simulink model "MicroMouseTemplate2"  (R2023a)
settings: Solver=FixedStepAuto  StartTime=0.0  StopTime=10.0  RelTol=1e-3  EnableMultiTasking=on
undefined symbols (not defined in the file): samplingTime
settings Model: STM32="{\"DigitalPortWrite\":[{\"ID\":\"MicroMouseTemplate:84:3\"},{\"ID\":\"MicroMouseTemplate:84:4\"},{\"ID\":\"MicroMouseTemplate:84:5\"},{\"ID\":\"MicroMouseTemplate:84:6\"},{\"ID\":\"MicroMouseTemplate:84:7\"},{\"ID\":\"MicroMouseTemplate:84:8\"},{\"ID\":\"MicroMouseTemplate:84:9\"},{\"ID\":\"MicroMouseTemplate:84:10\"},{\"ID\":\"MicroMouseTemplate:160:19\"},{\"ID\":\"MicroMouseTemplate:2479:4\"},{\"ID\":\"MicroMouseTemplate:2479:6\"},{\"ID\":\"MicroMouseTemplate:2479:7\"},{\"ID\":\"MicroMouseTemplate:2479:8\"},{\"ID\":\"MicroMouseTemplate2:84:3\"},{\"ID\":\"MicroMouseTemplate2:84:4\"},{\"ID\":\"MicroMouseTemplate2:84:5\"},{\"ID\":\"MicroMouseTemplate2:84:6\"},{\"ID\":\"MicroMouseTemplate2:84:7\"},{\"ID\":\"MicroMouseTemplate2:84:8\"},{\"ID\":\"MicroMouseTemplate2:84:9\"},{\"ID\":\"MicroMouseTemplate2:84:10\"},{\"ID\":\"MicroMouseTemplate2:160:19\"},{\"ID\":\"MicroMouseTemplate2:2479:4\"},{\"ID\":\"MicroMouseTemplate2:2479:6\"},{\"ID\":\"MicroMouseTemplate2:2479:7\"},{\"ID\":\"MicroMouseTemplate2:2479:8\"}],\"PWMOutput\":[{\"ID\":\"MicroMouseTemplate:160:24\"},{\"ID\":\"MicroMouseTemplate:160:25\"},{\"ID\":\"MicroMouseTemplate2:160:24\"},{\"ID\":\"MicroMouseTemplate2:160:25\"}],\"AnalogInput\":[{\"ID\":\"MicroMouseTemplate:2357:1\"},{\"ID\":\"MicroMouseTemplate2:2357:1\"}],\"DigitalPortRead\":[{\"ID\":\"MicroMouseTemplate:2483:3\"},{\"ID\":\"MicroMouseTemplate:2483:4\"},{\"ID\":\"MicroMouseTemplate2:2483:3\"},{\"ID\":\"MicroMouseTemplate2:2483:4\"}]}"  SimulationMode=external  ExtModeTrigDuration=10  Creator=JesseJabezArendse  LastModifiedBy=khanm
settings SolverCC: AllowMultiTaskInputOutput=on  AutoInsertRateTranBlk=on  InsertRTBMode=Never (minimum delay)
settings OptimizationCC: EnhancedBackFolding=on  PassReuseOutputArgsAs=Individual arguments  StateBitsets=on  DataBitsets=on  ZeroExternalMemoryAtStartup=off  ZeroInternalMemoryAtStartup=off  NoFixptDivByZeroProtection=on  MaxStackSize=64  OptimizeBlockOrder=speed  DifferentSizesBufferReuse=on  EfficientTunableParamExpr=on
settings DebuggingCC: MultiTaskCondExecSysMsg=none  ParameterOverflowMsg=none  ParameterPrecisionLossMsg=none  ParameterTunabilityLossMsg=error
settings HardwareCC: ProdBitPerPointer=32  ProdBitPerSizeT=32  ProdBitPerPtrDiffT=32  ProdLargestAtomicInteger=Long  ProdLargestAtomicFloat=Double  ProdWordSize=32  ProdLongLongMode=on  ProdHWDeviceType=ARM Compatible->ARM Cortex  TargetBitPerPointer=64  TargetBitPerSizeT=64  TargetBitPerPtrDiffT=64  TargetLongLongMode=on  TargetIntDivRoundTo=Zero  TargetEndianess=LittleEndian  TargetWordSize=64  TargetHWDeviceType=MATLAB Host
settings ModelReferenceCC: EnableParallelModelReferenceBuilds=on  ParallelModelReferenceMATLABWorkerInit=Copy Base Workspace  SupportModelReferenceSimTargetCustomCode=on
settings SFSimCC: MATLABDynamicMemAlloc=off  SimHardwareAcceleration=native
settings RTWCC: Description=Embedded Coder  SystemTargetFile=ert.tlc  HardwareBoard=STM32L4xx Based  TLCOptions=-p0 -aInlineSetEventsForThisBaseRateFcn=TLC_FALSE -aSuppressMultiTaskScheduler=TLC_FALSE -aRateBasedStepFcn=1  TemplateMakefile=ert_default_tmf  Toolchain=GNU Tools for ARM Embedded Processors  CodeExecutionProfiling=on  CodeProfilingInstrumentation=coarse
settings RTWCC: CustomHeaderCode=|
  | #include "MicroMouseProgramming\Core\Inc\IMU.h"
  | #include "MicroMouseProgramming\Core\Inc\CustomWhile.h"
  | #include "MicroMouseProgramming\Core\Inc\Motors.h"
settings RTWCC: CustomInclude=|
  | MicroMouseProgramming\Core\Inc\
  | MicroMouseProgramming\Core\Src\
settings RTWCC: CustomSource=|
  | MicroMouseProgramming\Core\Src\IMU.c
  | MicroMouseProgramming\Core\Src\CustomWhile.c
  | MicroMouseProgramming\Core\Src\Motors.c
settings CodeAppCC: ForceParamTrailComments=on  IgnoreCustomStorageClasses=off  OperatorAnnotations=on  SimulinkDataObjDesc=on  SFDataObjDesc=on  InsertBlockDesc=on
settings ERTTargetCC: CodeReplacementLibrary=ARM Cortex-M  SupportNonFinite=off  SupportComplex=off  ExtModeTransport=3  ExtModeStaticAlloc=on  ExtModeStaticAllocSize=2048  ExtModeMexFile=ext_xcp  ExtModeIntrfLevel=Level2 - Open

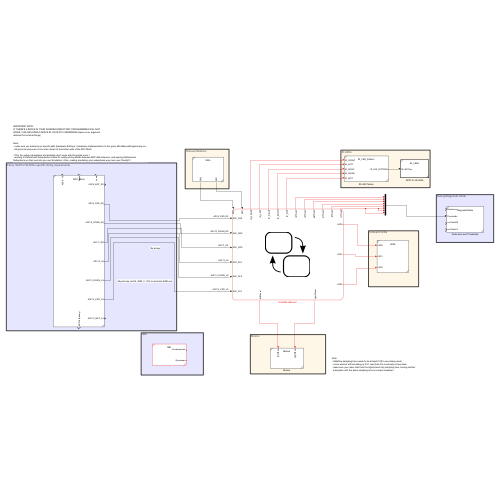
[thumbnail: Simulink's stored preview of the top-level diagram]
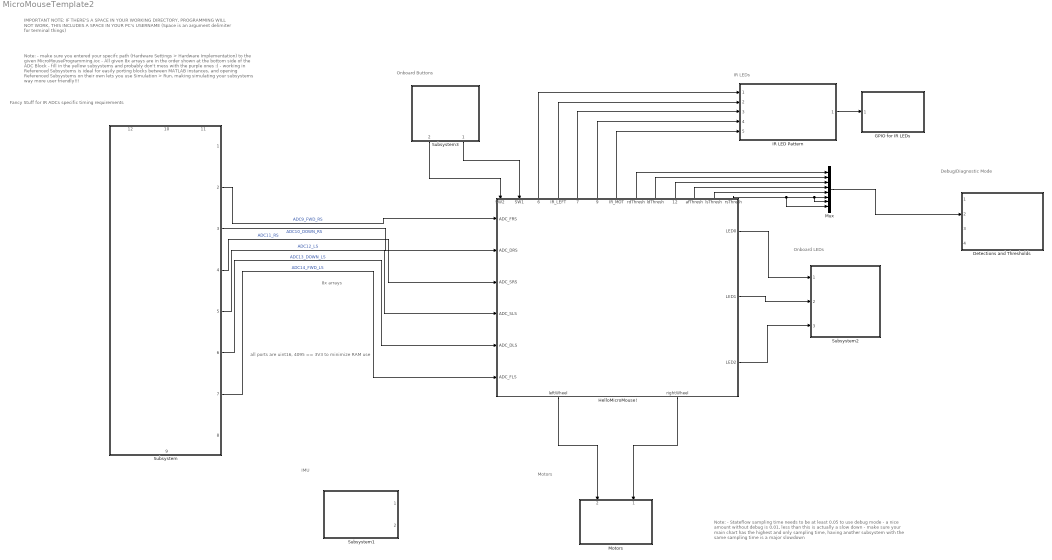
== system MicroMouseTemplate2 ==
  note: IMPORTANT NOTE:
      | IF THERE'S A SPACE IN YOUR WORKING DIRECTORY, PROGRAMMING WILL NOT WORK, THIS INCLUDES A SPACE IN YOUR PC's USERNAME (Space is an argument delimiter for terminal things)
  note: Note:
      | - make sure you entered your specifc path (Hardware Settings > Hardware Implementation) to the given MicroMouseProgramming.ioc
      | - All given 8x arrays are in the order shown at the bottom side of the ADC Block
      |
      | - fill in the yellow subsystems and probably don't mess with the purple ones :)
      | - working in Referenced Subsystems is ideal for easily porting blocks between MATLAB instances, and opening Referenced Subsystems on their own lets you use Simulation > Run, making simulating your subsystems way more user friendly!!!
  note: 8x arrays
  note: all ports are uint16, 4095 == 3V3 to minimize RAM use
  note: IMU
  note: Note:
      | - Stateflow sampling time needs to be at least 0.05 to use debug mode
      | - a nice amount without debug is 0.01, less than this is actually a slow down
      | - make sure your main chart has the highest and only sampling time, having another
      | subsystem with the same sampling time is a major slowdown
  note: Fancy Stuff for IR ADCs specific timing requirements
  note: IR LEDs
  note: Motors
  note: Onboard Buttons
  note: Onboard LEDs
  note: Debug/Diagnostic Mode
  Detections and Thresholds : Subsystem  ReferencedSubsystem=DiagnosticMode
  GPIO for IR LEDs : Subsystem  TreatAsAtomicUnit=on  SystemSampleTime=samplingTime  ReferencedSubsystem=IR_LEDs
  HelloMicroMouse! : Stateflow chart  TreatAsAtomicUnit=on
      settings: PortSchema="{\"entries\":[{\"content\":{\"sides\":[{\"content\":{\"connectorIds\":[\"In6\",\"In3\",\"In8\",\"In7\",\"In4\",\"In5\"]},\"type\":\"ConnectorPlacement.EquallySpacedRectSide\",\"uuid\":\"f52daa4f-6374-42e5-9ef1-0ccc99d09b58\"},{\"content\":{\"connectorIds\":[\"Out1\",\"Out4\",\"Out5\"],\"side\":\"RIGHT\"},\"type\":\"ConnectorPlacement.EquallySpacedRectSide\",\"uuid\":\"94b478cc-4dde-45c7-a588-77cf2b43cdb7\"},{\"content\":{\"connectorIds\":[\"In1\",\"In2\",\"Out6\",\"Out8\",\"Out7\",\"Out9\",\"Out16\",\"Out10\",\"Out11\",\"Out12\",\"Out13\",\"Out14\",\"Out15\"],\"side\":\"TOP\"},\"type\":\"ConnectorPlacement.EquallySpacedRectSide\",\"uuid\":\"afff2079-ea5c-423e-9722-09c3bbce433b\"},{\"content\":{\"connectorIds\":[\"Out2\",\"Out3\"],\"side\":\"BOTTOM\"},\"type\":\"ConnectorPlacement.EquallySpacedRectSide\",\"uuid\":\"94e93a1d-795d-41a3-b2d8-d520b2bf47ef\"}]},\"type\":\"ConnectorPlacement.EquallySpacedConnector\",\"uuid\":\"d4d35636-54af-48ac-af70-d56caef5e090\"}],\"packageUris\":[\"http://schema.mathworks.com/mf0/Connector/R2020b\"],\"version\":\"1.0\"}"
  IR LED Pattern : Subsystem  ReferencedSubsystem=IR_LED_Pattern
  Motors : Subsystem  ReferencedSubsystem=Motors
      settings: PortSchema="{\"entries\":[{\"content\":{\"sides\":[{\"content\":{},\"type\":\"ConnectorPlacement.EquallySpacedRectSide\",\"uuid\":\"c0768360-d607-41d7-924d-4f6c7a7c5513\"},{\"content\":{\"side\":\"RIGHT\"},\"type\":\"ConnectorPlacement.EquallySpacedRectSide\",\"uuid\":\"76549d19-b608-4a9d-9981-587ff77a2575\"},{\"content\":{\"connectorIds\":[\"In2\",\"In1\"],\"side\":\"TOP\"},\"type\":\"ConnectorPlacement.EquallySpacedRectSide\",\"uuid\":\"f7c4009a-c050-4e8b-9774-5a337efc0393\"}]},\"type\":\"ConnectorPlacement.EquallySpacedConnector\",\"uuid\":\"93b2f239-44e8-47ae-a398-357dc23e174c\"}],\"packageUris\":[\"http://schema.mathworks.com/mf0/Connector/R2020b\"],\"version\":\"1.0\"}"
  Mux : Mux  Inputs=8
  Subsystem : Subsystem  ReferencedSubsystem=ADC_Block
      settings: PortSchema="{\"entries\":[{\"content\":{\"sides\":[{\"content\":{},\"type\":\"ConnectorPlacement.EquallySpacedRectSide\",\"uuid\":\"be6b81d5-7a49-4e34-b35f-0c07892094fc\"},{\"content\":{\"connectorIds\":[\"Out1\",\"Out2\",\"Out3\",\"Out4\",\"Out5\",\"Out6\",\"Out7\",\"Out8\"],\"side\":\"RIGHT\"},\"type\":\"ConnectorPlacement.EquallySpacedRectSide\",\"uuid\":\"5e22590a-b7c0-4c63-8de4-8d81fd6c3849\"},{\"content\":{\"connectorIds\":[\"Out12\",\"Out10\",\"Out11\"],\"side\":\"TOP\"},\"type\":\"ConnectorPlacement.EquallySpacedRectSide\",\"uuid\":\"da97636e-cea0-4a10-8fe5-d807f9ee999f\"},{\"content\":{\"connectorIds\":[\"Out9\"],\"side\":\"BOTTOM\"},\"type\":\"ConnectorPlacement.EquallySpacedRectSide\",\"uuid\":\"a593d780-81a8-4730-a8bc-2bbf356cafe4\"}]},\"type\":\"ConnectorPlacement.EquallySpacedConnector\",\"uuid\":\"0bcac921-e51a-4437-9183-315712d0a8c2\"}],\"packageUris\":[\"http://schema.mathworks.com/mf0/Connector/R2020b\"],\"version\":\"1.0\"}"
  Subsystem1 : Subsystem  ReferencedSubsystem=IMU
  Subsystem2 : Subsystem  ReferencedSubsystem=LEDs
  Subsystem3 : Subsystem  ReferencedSubsystem=SWs
      settings: PortSchema="{\"entries\":[{\"content\":{\"sides\":[{\"content\":{},\"type\":\"ConnectorPlacement.EquallySpacedRectSide\",\"uuid\":\"525c1d33-3535-4f4c-aa7a-529c732595a4\"},{\"content\":{\"side\":\"RIGHT\"},\"type\":\"ConnectorPlacement.EquallySpacedRectSide\",\"uuid\":\"892b90bb-1dbb-40cd-aa67-d09788eff32d\"},{\"content\":{\"side\":\"TOP\"},\"type\":\"ConnectorPlacement.EquallySpacedRectSide\",\"uuid\":\"6623a0d6-78eb-4978-b109-dfe6d3d1ab9b\"},{\"content\":{\"connectorIds\":[\"Out2\",\"Out1\"],\"side\":\"BOTTOM\"},\"type\":\"ConnectorPlacement.EquallySpacedRectSide\",\"uuid\":\"a7ac3c79-7bca-470d-bb1f-b760bc3a3657\"}]},\"type\":\"ConnectorPlacement.EquallySpacedConnector\",\"uuid\":\"47292853-ce7e-4392-82cf-216c29274acb\"}],\"packageUris\":[\"http://schema.mathworks.com/mf0/Connector/R2020b\"],\"version\":\"1.0\"}"
  wires:
  Subsystem3/1 -> HelloMicroMouse!/2(SW1)
  Subsystem3/2 -> HelloMicroMouse!/1(SW2)
  HelloMicroMouse!/1(LED0) -> Subsystem2/1
  IR LED Pattern/1 -> GPIO for IR LEDs/1
  Subsystem/6 -> HelloMicroMouse!/4(ADC_DLS)  "ADC13_DOWN_LS"
  Subsystem/3 -> HelloMicroMouse!/3(ADC_DRS)  "ADC10_DOWN_RS"
  HelloMicroMouse!/2(leftWheel) -> Motors/2
  HelloMicroMouse!/3(rightWheel) -> Motors/1
  HelloMicroMouse!/5(LED2) -> Subsystem2/3
  HelloMicroMouse!/4(LED1) -> Subsystem2/2
  Subsystem/2 -> HelloMicroMouse!/6(ADC_FRS)  "ADC9_FWD_RS"
  Subsystem/7 -> HelloMicroMouse!/5(ADC_FLS)  "ADC14_FWD_LS"
  Subsystem/5 -> HelloMicroMouse!/7(ADC_SLS)  "ADC12_LS"
  Subsystem/4 -> HelloMicroMouse!/8(ADC_SRS)  "ADC11_RS"
  HelloMicroMouse!/6(IR_FRONT) -> IR LED Pattern/1
  HelloMicroMouse!/8(IR_LEFT) -> IR LED Pattern/2
  HelloMicroMouse!/7(IR_RIGHT) -> IR LED Pattern/3
  HelloMicroMouse!/9(IR_DOWN) -> IR LED Pattern/4
  HelloMicroMouse!/10(rdThresh) -> Mux/1
  HelloMicroMouse!/11(ldThresh) -> Mux/2
  HelloMicroMouse!/12(adThresh) -> Mux/3
  HelloMicroMouse!/13(afThresh) -> Mux/4
  HelloMicroMouse!/14(lsThresh) -> Mux/5
  Mux/1 -> Detections and Thresholds/2
  HelloMicroMouse!/15(rsThresh) -> Mux/8, Mux/7, Mux/6
  HelloMicroMouse!/16(IR_MOT) -> IR LED Pattern/5

== stateflow chart MicroMouseTemplate2/HelloMicroMouse! ==
  state Callibrate
    entry:
    complete = 0;
    during:
    LED0 = false;
    LED1 = ~LED1;
    state RotateTo270
      during:
      leftWheel = -77;
      rightWheel = 77;
      on after(delay ,sec):
      leftWheel = 0;
      rightWheel = 0;
      if ADC_SRS > noWallAmbRS
      noWallAmbRS = ADC_SRS;
      end
      on after(1.7,sec):
      IR_RIGHT = 1;
      if ADC_SRS > noWallRS
      noWallRS = ADC_SRS;
      end
      on after(2.6,sec):
      IR_RIGHT = 0;
      complete = 1;
      exit:
      %Adjusts thresholds based on ambient light
      noWallRS = noWallRS -noWallAmbRS
    state RotateTo90
      during:
      leftWheel = -77;
      rightWheel = 77;
      on after(delay ,sec):
      leftWheel = 0;
      rightWheel = 0;
      if ADC_SLS > noWallAmbLS
      noWallAmbLS = ADC_SLS;
      end
      on after(1.7,sec):
      IR_LEFT = 1;
      if ADC_SLS > noWallLS
      noWallLS = ADC_SLS;
      end
      on after(2.6,sec):
      IR_LEFT = 0;
      complete = 1;
      exit:
      %Adjusts thresholds based on ambient light
      noWallLS = noWallLS -noWallAmbLS
    state RotateTo360
      entry:
      complete = 0;
      during:
      leftWheel = -77;
      rightWheel = 77;
      on after(delay,sec):
      leftWheel = 0;
      rightWheel = 0;
      on after(1.8,sec):
      if (ADC_DRS+ADC_DLS)/2 > adThresh
      adThresh = (ADC_DRS+ADC_DLS)/2 ;
      end
      on after(2.2,sec):
      if (ADC_DLS) > rdThresh
      rdThresh = ADC_DLS;
      end
      if (ADC_DRS) > ldThresh
      ldThresh = ADC_DRS;
      end
      complete =1;
      exit:
      adThresh = adThresh-200;
      rdThresh = rdThresh+600;
      ldThresh = ldThresh+600;
      rsThresh = (rsThresh + noWallRS)/2;
      lsThresh = (lsThresh + noWallLS)/2;
    state RotateTo180
      entry:
      complete = 0;
      during:
      leftWheel = -77;
      rightWheel = 77;
      on after(delay ,sec):
      leftWheel = 0;
      rightWheel = 0;
      IR_FRONT = 1;
      on after(1.8,sec):
      if (ADC_FRS+ADC_FLS)/2 > afThresh
      afThresh = (ADC_FRS+ADC_FLS)/2;
      end
      on after(2.2,sec):
      IR_FRONT = 0;
      IR_LEFT = 1;
      IR_RIGHT = 1;
      if ADC_SLS > lsThresh
      lsThresh = ADC_SLS;
      end
      if ADC_SRS > rsThresh
      rsThresh = ADC_SRS;
      end
      on after(2.6,sec):
      IR_LEFT = 0;
      IR_RIGHT = 0;
      complete = 1;
    state CheckAmbience
      entry:
      complete = 0
      during:
      if (ADC_FRS+ADC_FLS)/2 > ambF
      ambF = (ADC_FRS+ADC_FLS)/2; %get maximum ambient light
      end
      if ADC_SLS > ambLS
      ambLS = ADC_SRS;
      end
      if ADC_SRS > ambRS
      ambRS = ADC_SRS;
      end
      on after(1,sec):
      complete = 1;
      exit:
      %Adjusts thresholds based on ambient light
      afThresh = afThresh - ambF;
      rsThresh = rsThresh - ambRS;
      lsThresh = lsThresh - ambLS;
    (default) -> RotateTo90
    RotateTo270 -> RotateTo360 : [complete == 1]
    RotateTo90 -> RotateTo180 : [complete==1]
    CheckAmbience -> RotateTo270 : [complete==1]
    RotateTo180 -> CheckAmbience : [complete==1]
  state Adjust
    state Turn
      entry:
      complete = 0;
      note: Do not put any code along
          | the transitions that run
          | down the right side!
      (default) -> (junction 299)
      (junction 299) -> (junction 300) [order 1] : [ff == 1 && rf == 1 && lf == 1]
      (junction 299) -> (junction 303) [order 2]
      (junction 300) -> (junction 301) : {delay = 2.2,leftWheel = 77, rightWheel = -77}
      (junction 301) -> (junction 302)
      (junction 302) -> (junction 306)
      (junction 303) -> (junction 304) [order 1] : [ff ==1 && rf==1 ]
      (junction 303) -> (junction 307) [order 2]
      (junction 304) -> (junction 305) : {delay = 1,rightWheel=77,leftWheel = -77}
      (junction 305) -> (junction 306)
      (junction 306) -> (junction 310)
      (junction 307) -> (junction 308) [order 1] : [ff ==1 && lf == 1]
      (junction 307) -> (junction 311) [order 2]
      (junction 308) -> (junction 309) : {delay = 1,rightWheel=77,leftWheel = -77}
      (junction 309) -> (junction 310)
      (junction 310) -> (junction 314)
      (junction 311) -> (junction 312) [order 1] : [ff == 1]
      (junction 311) -> (junction 315) [order 2] : {leftWheel = 77, rightWheel=77}
      (junction 312) -> (junction 313) : {delay = 1 ,rightWheel=77,leftWheel = -77}
      (junction 313) -> (junction 314)
      (junction 314) -> (junction 319)
      (junction 316) -> (junction 315)
      (junction 319) -> (junction 316)
      (junction 315) -> (junction 317) : {complete =1}
    state SlightRight
      during:
      LED2 = false;
      LED1 = false;
      LED0 = true;
      leftWheel = 85;
      rightWheel = 75;
    state CheckWalls
      entry:
      leftWheel =0;
      rightWheel = 0;
      LED0 = false;
      LED1 = false;
      LED2 = false;
      IR_DOWN = 0;
      exit:
      IR_DOWN = 1;
      state CheckLeft
        entry:
        complete = 0;
        wallAmb = 0;
        wallDet = 0;
        during:
        if ADC_SRS > wallAmb
        wallAmb = ADC_SRS;
        end
        on after(0.3,sec):
        IR_RIGHT = 1;
        if ADC_SRS > wallDet
        wallDet = ADC_SRS;
        end
        on after(0.6,sec):
        IR_RIGHT = 0;
        wallDet = wallDet - wallAmb;
        if wallDet>rsThresh
        lf = 1;%left flag
        LED0 = true;
        end
        on after(0.9,sec):
        complete = 1;
      state CheckRight
        entry:
        complete = 0;
        wallAmb = 0;
        wallDet = 0;
        during:
        if ADC_SLS > wallAmb
        wallAmb = ADC_SLS;
        end
        on after(0.3,sec):
        IR_LEFT = 1;
        if ADC_SLS > wallDet
        wallDet = ADC_SLS;
        end
        on after(0.6,sec):
        IR_LEFT = 0;
        wallDet = wallDet - wallAmb;
        if wallDet>lsThresh
        rf = 1;%left flag
        LED2 = true;
        end
        on after(0.9,sec):
        complete = 1
      state CheckFront
        entry:
        IR_FRONT = 1;
        during:
        if (ADC_FRS+ADC_FLS)/2>afThresh
        ff = 1;%front flag
        LED1 = true;
        end
        exit:
        IR_FRONT = 0;
      (default) -> CheckLeft
      CheckRight -> CheckFront : [complete==1]
      CheckLeft -> CheckRight : [complete==1]
    state GoStraight
      during:
      LED1 = true;
      LED0 = false;
      LED2 = false;
      leftWheel = 80;
      rightWheel = 80;
    state WaitForTurn
      entry:
      complete = 0;
      on after(delay,sec):
      leftWheel = 0;
      rightWheel = 0;
      complete = 1;
      exit:
      lf = 0;
      rf = 0;
      ff = 0;
    state SlightLeft
      during:
      LED0 = false;%take note of flip
      LED1 = false;
      LED2 = true;
      leftWheel = 75;
      rightWheel = 85;
    (default) -> GoStraight
    SlightRight -> GoStraight [order 1] : [ADC_DRS < ldThresh]{leftWheel = 75; rightWheel = 75}
    GoStraight -> SlightRight [order 3] : [ADC_DRS > ldThresh]{leftWheel = 75; rightWheel = 75}
    SlightRight -> CheckWalls [order 2] : [(ADC_DLS+ADC_DRS)/2 < adThresh]{leftWheel = 0,rightWheel = 0}
    GoStraight -> CheckWalls [order 1] : [(ADC_DLS+ADC_DRS)/2 < adThresh]{leftWheel = 0,rightWheel = 0}
    CheckFront -> Turn : after(0.3,sec)
    SlightLeft -> CheckWalls [order 1] : [(ADC_DLS+ADC_DRS)/2 < adThresh]{leftWheel = 0,rightWheel = 0}
    Turn -> WaitForTurn : [complete == 1]
    GoStraight -> SlightLeft [order 2] : [ADC_DLS > rdThresh]{leftWheel = 75; rightWheel = 75}
    SlightLeft -> GoStraight [order 2] : [ADC_DLS < rdThresh]{leftWheel = 75; rightWheel = 75}
    WaitForTurn -> (junction 325) : [complete == 1]
    (junction 325) -> GoStraight
  state WaitUntilButtonPressed
    during:
    LED0 = ~LED0;
    %set IRS
    IR_FRONT = 0;
    IR_LEFT = 0;
    IR_RIGHT = 0;
    IR_MOT = 0;
    IR_DOWN = 0 ;
    %set init flags
    lf = 0;
    rf = 0;
    ff = 0;
    %set thresholds
    rsThresh = l;
    lsThresh = l;
    afThresh = l;
    adThresh = l;
    ldThresh = l;
    rdThresh = l;
    ambRS = l;
    ambLS=l;
    ambF=l;
    noWallLS=l;
    noWallRS=l;
    noWallAmbLS=l;
    noWallAmbRS=l;
    wallDet = l;
    wallAmb = l;
    delay = 1;
  state StopAll
    entry:
    LED0 = false;
    LED1 = false;
    LED2 = false;
    leftWheel = 0;
    rightWheel = 0;
  RotateTo360 -> Adjust : [complete == 1]
  (default) -> WaitUntilButtonPressed
  WaitUntilButtonPressed -> Callibrate : [SW2 ]
  Adjust -> StopAll : [SW2]
  data: SW2 input; LED0 output; SW1 input; leftWheel output int8; rightWheel output int8; ADC_DRS input; ADC_DLS input; LED1 output; LED2 output; ADC_FLS input; ADC_FRS input; ADC_SLS input; ADC_SRS input; IR_FRONT output; IR_RIGHT output; IR_LEFT output; IR_DOWN output; complete local; lf local; ff local; rf local; delay local; rdThresh output; ldThresh output; adThresh output; afThresh output; lsThresh output; rsThresh output; l local uint16 =0; IR_MOT output; ambF local; ambLS local; ambRS local; noWallAmbLS local; noWallAmbRS local; noWallLS local; noWallRS local; wallAmb local; wallDet local
